simulink model "with_regulation"  (R2017b)
settings: Solver=ode23tb  StartTime=0.0  StopTime=20  RelTol=1e-4  EnableMultiTasking=on
libraries: powerlib x4, electricdrivelib x2, simulink x1
Description:
  | Copyright 2008-2017 The MathWorks, Inc.
settings Model: NumberOfSteps=1000  Creator=MathWorks  LastModifiedBy=carter trautmann
settings DataIOCC: LimitDataPoints=on  SaveFormat=Array  SignalLoggingSaveFormat=ModelDataLogs
settings OptimizationCC: ExpressionDepthLimit=2147483647  InitFltsAndDblsToZero=on  EfficientMapNaN2IntZero=off  LifeSpan=inf
settings DebuggingCC: SaveWithParameterizedLinksMsg=none  UnderspecifiedInitializationDetection=Classic  MergeDetectMultiDrivingBlocksExec=none  FcnCallInpInsideContextMsg=warning  AllowSymbolicDim=off  StateNameClashWarn=warning  SFUnexpectedBacktrackingDiag=warning  SFNoUnconditionalDefaultTransitionDiag=warning  SFExecutionAtInitializationDiag=none
settings HardwareCC: ProdBitPerPointer=32  ProdBitPerSizeT=32  ProdBitPerPtrDiffT=32  ProdLargestAtomicFloat=None  ProdIntDivRoundTo=Undefined  ProdEndianess=Unspecified  ProdWordSize=32  ProdHWDeviceType=32-bit Generic
settings ModelReferenceCC: PropagateSignalLabelsOutOfModel=off
settings CodeAppCC: StateflowObjectComments=on
settings GRTTargetCC: TargetFcnLib=ansi_tfl_tmw.mat  TargetLangStandard=C89/C90 (ANSI)  GeneratePreprocessorConditionals=Disable all  CombineOutputUpdateFcns=off  GRTInterface=on
settings ConfigComp: CovMetricSettings=dw  CovHtmlReporting=on  CovSaveCumulativeToWorkspaceVar=on  CovSaveSingleToWorkspaceVar=on  CovExternalEMLEnable=off  CovSFcnEnable=off
settings SimscapeCC: SimscapeNormalizeSystem=off

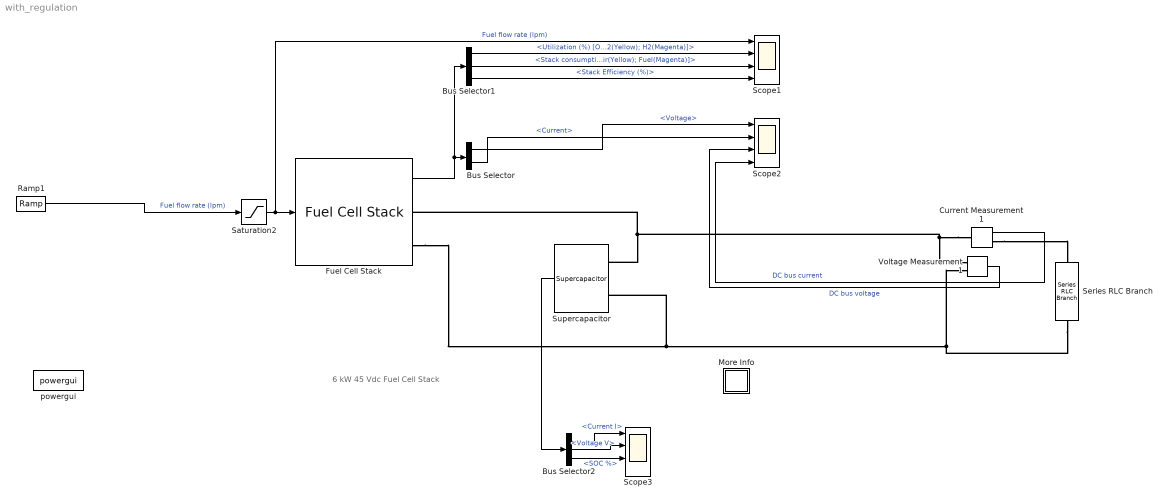
== system with_regulation ==
  note: 6 kW 45 Vdc Fuel Cell Stack
  Bus Selector : BusSelector  OutputSignals=Voltage,Current
  Bus Selector1 : BusSelector  OutputSignals=Utilization (%) [O2(Yellow); H2(Magenta)],Stack consumption (lpm) [Air(Yellow); Fuel(Magenta)],Stack Efficiency (%)
  Bus Selector2 : BusSelector  OutputSignals=Current I,Voltage V,SOC %
  Current Measurement1 : powerlib/Measurements/Current Measurement  PhasorSimulation=off  OutputType=Complex  PSBequivalent=0
  Fuel Cell Stack : electricdrivelib/Extra Sources/Fuel Cell Stack  PresetModel=No (User-Defined)  FcType=Proton Exchange Membrane (PEM)  Detailed=Detailed  Eoc="[43  40]"  NomVI="[10            35]"  EndVI="[75   23]"  Nc=46  n=60  TOp=65  AirFr=175  SuppPress="[0.4           1]"  Comp="[99.95           21            1]"  SignX=off  SignY=off  FlowRateH2=on  FlowRateAir=off  SystemTemp=off  SystemPH2=off  SystemPAir=off  FCDyn=off  FC_tau=0  Peak_O2=80  V_Under=10
      settings: SourceProductName=Simscape Power Systems  SourceProductBaseCode=PS
  More Info : Subsystem
      settings: OpenFcn=showdemo(bdroot(gcb))
      mask Display: disp('?')
  Ramp1 : simulink/Sources/Ramp  slope=10  start=1  X0=0
  Saturation2 : Saturate  UpperLimit=85  LowerLimit=0
  Scope1 : Scope  NumInputPorts=4
  Scope2 : Scope  NumInputPorts=4
  Scope3 : Scope  NumInputPorts=4
  Series RLC Branch : powerlib/Elements/Series RLC Branch  LConnTagsString=__new0  RConnTagsString=__new0  BranchType=RL  Resistance=100  Inductance=100  SetiL0=off  InitialCurrent=0  Capacitance=1e-6  Setx0=off  InitialVoltage=0  Measurements=None
  Supercapacitor : electricdrivelib/Extra Sources/Supercapacitor  C=19.3  Rdc=8.9e-3  Voltage=48  Ns=3  Np=1  Vinit=0  Temp=25  PresetModel=off  EstParam=off  Nc=1  r=1e-9  epsilon=6.0208e-10  Ich=10  Vstern="[0.161  2.7  7.8]"  Self_dis=on  Ioc=10  Vself="[48  47.8  47.06  44.65]"  demandeplot=off  I="[10  20 100  500]"  Units=sec  Vmax=0  If=0  deltaV=0  alpha=0  sec=0
      settings: SourceProductName=Simscape Power Systems  SourceProductBaseCode=PS
  Voltage Measurement1 : powerlib/Measurements/Voltage Measurement  PhasorSimulation=off  OutputType=Complex  PSBequivalent=0
  powergui : powerlib/powergui  SimulationMode=Continuous  SampleTime=1e-6  frequency=60  Iterations=50  frequencyindice=0  Pbase=100e6  ErrMax=1e-4  UnitsV=kV  UnitsW=MW  buscounter=0  FunctionMessages=off  echomessages=off  EnableUseOfTLC=off  CurrentSourceSwitches=off  DisableSnubberDevices=off  DisableRonSwitches=off  DisableVfSwitches=off  DisplayEquations=off  SolverType=Tustin  Interpol=off  ExternalGateDelay=off  methode=off  Ts=0  x0status=blocks  SPID=off  SwTol=0  HookPort=off  RestoreLinks=warning  ResistiveCurrentMeasurement=off  Frange=[0:2:500]  Ylog=off  Xlog=on  ShowGrid=off  save=off  variable=ZData  structure=0  ZoomFFT=on  StartTime=0.0  cycles=1  DisplayStyle=1  fundamental=60  FreqAxis=off  MaxFrequency=1000  frequencyindicesteady=1  RmsSteady=1  display=off
  wires:
  Fuel Cell Stack/1 -> Bus Selector1/1, Bus Selector/1
  Bus Selector/1 -> Scope2/1  "<Voltage>"
  Bus Selector/2 -> Scope2/2  "<Current>"
  Voltage Measurement1/1 -> Scope2/3  "DC bus voltage"
  Current Measurement1/1 -> Scope2/4  "DC bus current"
  Bus Selector1/1 -> Scope1/2  "<Utilization (%) [O2(Yellow); H2(Magenta)]>"
  Bus Selector1/3 -> Scope1/4  "<Stack Efficiency (%)>"
  Bus Selector1/2 -> Scope1/3  "<Stack consumption (lpm) [Air(Yellow); Fuel(Magenta)]>"
  Ramp1/1 -> Saturation2/1  "Fuel flow rate (lpm)"
  Saturation2/1 -> Fuel Cell Stack/1, Scope1/1  "Fuel flow rate (lpm)"
  Supercapacitor/1 -> Bus Selector2/1
  Bus Selector2/1 -> Scope3/1  "<Current I>"
  Bus Selector2/2 -> Scope3/2  "<Voltage V>"
  Bus Selector2/3 -> Scope3/3  "<SOC %>"
  connections:
  Series RLC Branch/RConn1 -- Supercapacitor/LConn2 -- Fuel Cell Stack/RConn2 -- Voltage Measurement1/LConn2
  Current Measurement1/RConn1 -- Series RLC Branch/LConn1
  Current Measurement1/LConn1 -- Supercapacitor/LConn1 -- Fuel Cell Stack/RConn1 -- Voltage Measurement1/LConn1

== system with_regulation/More Info ==
